simulink model "sl_GDT_RRR"  (R2016b)
settings: Solver=ode45  StartTime=0.0  StopTime=t_sim  MaxStep=1e-3  RelTol=1e-8  EnableMultiTasking=on
values from neighbouring files (symbols this model uses):
  n_ptos = 4    [DEFENSA_PRUEBASgraficas.m]    (also in GDT_C_RRR.m = in(10); GDT_Lineal_trap.m; GDT_RRR.m = in(7))
  t_init = 2    [DEFENSA_PRUEBASgraficas.m]    (also in GDT_C_RRR.m = in(11); GDT_Lineal_trap.m; GDT_RRR.m = in(8))
  t_tray = 1    [DEFENSA_PRUEBASgraficas.m]    (also in GDT_C_RRR.m = in(12); GDT_Lineal_trap.m; GDT_RRR.m = in(9))
  xyz_fin = CinematicaDirecta([pi/2;pi/3;-pi/3])    [DEFENSA_PRUEBASgraficas.m]    (also in GDT_Lineal_trap.m)
  xyz_init = CinematicaDirecta([0;pi/4;-pi/4])    [DEFENSA_PRUEBASgraficas.m]    (also in GDT_Lineal_trap.m)
settings Model: ExtModeTrigMode=oneshot  ExtModeArmWhenConnect=off  Creator=Manuel G. Ortega  LastModifiedBy=Daniel
settings DataIOCC: SaveFormat=Array  SignalLoggingSaveFormat=ModelDataLogs
settings OptimizationCC: BooleanDataType=off  ExpressionDepthLimit=2147483647  InitFltsAndDblsToZero=on  LifeSpan=inf
settings DebuggingCC: SaveWithParameterizedLinksMsg=none  UnderspecifiedInitializationDetection=Classic  MergeDetectMultiDrivingBlocksExec=none  SignalResolutionControl=TryResolveAllWithWarning  MultiTaskDSMMsg=warning  MultiTaskCondExecSysMsg=none  FcnCallInpInsideContextMsg=warning  StateNameClashWarn=warning  SFUnexpectedBacktrackingDiag=warning  SFNoUnconditionalDefaultTransitionDiag=warning  SFExecutionAtInitializationDiag=none
settings HardwareCC: ProdBitPerPointer=32  ProdBitPerSizeT=32  ProdBitPerPtrDiffT=32  ProdLargestAtomicFloat=None  ProdIntDivRoundTo=Undefined  ProdEndianess=Unspecified  ProdWordSize=32  ProdHWDeviceType=32-bit Generic  TargetUnknown=on
settings ModelReferenceCC: PropagateSignalLabelsOutOfModel=off
settings GRTTargetCC: TargetFcnLib=ansi_tfl_tmw.mat  TargetLangStandard=C89/C90 (ANSI)  GeneratePreprocessorConditionals=Disable all  CombineOutputUpdateFcns=off  GRTInterface=on
settings ConfigComp: CovMetricSettings=dw  CovHtmlReporting=on  CovSaveCumulativeToWorkspaceVar=on  CovSaveSingleToWorkspaceVar=on  CovExternalEMLEnable=off  CovSFcnEnable=off

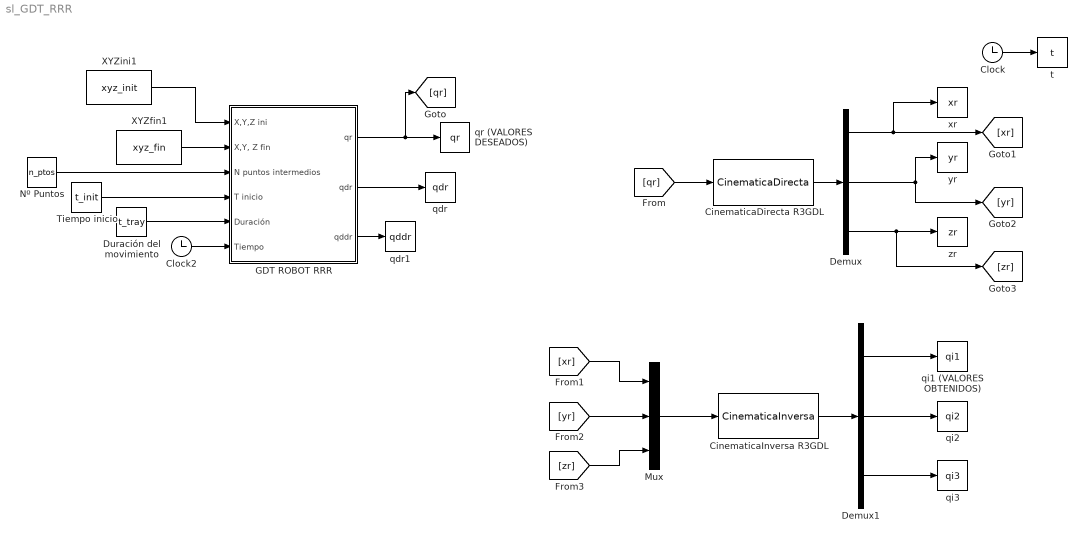
== system sl_GDT_RRR ==
  CinematicaDirecta R3GDL : MATLABFcn  MATLABFcn=CinematicaDirecta  OutputDimensions=3
  CinematicaInversa R3GDL : MATLABFcn  MATLABFcn=CinematicaInversa  OutputDimensions=3
  Clock : Clock
  Clock2 : Clock
  Demux : Demux  Outputs=3
  Demux1 : Demux  Outputs=3
  Duración del movimiento : Constant  Value=t_tray
  GDT ROBOT RRR : Subsystem
  Mux : Mux  Inputs=3
  Nº Puntos : Constant  Value=n_ptos
  Tiempo inicio : Constant  Value=t_init
  XYZfin1 : Constant  Value=xyz_fin
  XYZini1 : Constant  Value=xyz_init
  qdr : ToWorkspace  VariableName=qdr  SampleTime=-1
  qdr1 : ToWorkspace  VariableName=qddr  SampleTime=-1
  qi1 (VALORES OBTENIDOS) : ToWorkspace  VariableName=qi1  SampleTime=-1
  "qi2 " : ToWorkspace  VariableName=qi2  SampleTime=-1
  "qi3 " : ToWorkspace  VariableName=qi3  SampleTime=-1
  qr (VALORES DESEADOS) : ToWorkspace  VariableName=qr  SampleTime=-1
  t : ToWorkspace  VariableName=t  SampleTime=-1
  xr : ToWorkspace  VariableName=xr  SampleTime=-1
  yr : ToWorkspace  VariableName=yr  SampleTime=-1
  zr : ToWorkspace  VariableName=zr  SampleTime=-1
  wires:
  Clock/1 -> t/1
  Clock2/1 -> GDT ROBOT RRR/6(Tiempo)
  Duración del movimiento/1 -> GDT ROBOT RRR/5(Duración)
  Tiempo inicio/1 -> GDT ROBOT RRR/4(T inicio)
  Nº Puntos/1 -> GDT ROBOT RRR/3(N puntos intermedios)
  XYZfin1/1 -> GDT ROBOT RRR/2("X,Y, Z fin")
  XYZini1/1 -> GDT ROBOT RRR/1(X,Y,Z ini)
  GDT ROBOT RRR/1(qr) -> qr (VALORES DESEADOS)/1, [qr]
  [qr] -> CinematicaDirecta R3GDL/1
  CinematicaDirecta R3GDL/1 -> Demux/1
  Demux/1 -> xr/1, [xr]
  Demux/2 -> [yr], yr/1
  Demux/3 -> [zr], zr/1
  [yr] -> Mux/2
  [zr] -> Mux/3
  [xr] -> Mux/1
  Mux/1 -> CinematicaInversa R3GDL/1
  CinematicaInversa R3GDL/1 -> Demux1/1
  Demux1/1 -> qi1 (VALORES OBTENIDOS)/1
  Demux1/3 -> "qi3 "/1
  Demux1/2 -> "qi2 "/1
  GDT ROBOT RRR/2(qdr) -> qdr/1
  GDT ROBOT RRR/3(qddr) -> qdr1/1

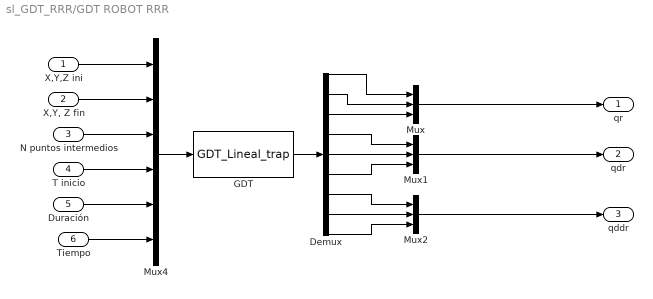
== system sl_GDT_RRR/GDT ROBOT RRR ==
  X,Y,Z ini : Inport
  "X,Y, Z fin" : Inport  Port=2
  N puntos intermedios : Inport  Port=3
  T inicio : Inport  Port=4
  Duración : Inport  Port=5
  Tiempo : Inport  Port=6
  Demux : Demux  Outputs=9
  "GDT " : MATLABFcn  MATLABFcn=GDT_Lineal_trap  OutputDimensions=9
  Mux : Mux  Inputs=3
  Mux1 : Mux  Inputs=3
  Mux2 : Mux  Inputs=3
  Mux4 : Mux  Inputs=6
  qr : Outport
  qdr : Outport  Port=2
  qddr : Outport  Port=3
  wires:
  Mux4/1 -> "GDT "/1
  X,Y,Z ini/1 -> Mux4/1
  "X,Y, Z fin"/1 -> Mux4/2
  N puntos intermedios/1 -> Mux4/3
  T inicio/1 -> Mux4/4
  Duración/1 -> Mux4/5
  Tiempo/1 -> Mux4/6
  "GDT "/1 -> Demux/1
  Mux/1 -> qr/1
  Demux/1 -> Mux/1
  Demux/2 -> Mux/2
  Demux/3 -> Mux/3
  Demux/5 -> Mux1/2
  Demux/4 -> Mux1/1
  Demux/6 -> Mux1/3
  Mux1/1 -> qdr/1
  Demux/8 -> Mux2/2
  Mux2/1 -> qddr/1
  Demux/7 -> Mux2/1
  Demux/9 -> Mux2/3
